simulink model "PassengerCar"  (R2019b)
settings: Solver=ode1  StartTime=0  StopTime=25  FixedStep=1.0000000000000000e-003  RelTol=1e-3
InitFcn:
  | sampleTime = str2double(get_param(bdroot, 'FixedStep'));
undefined symbols (not defined in the file or in its folder): AccPedalPos, BrakePedalPos, BrakeSwitch, DiscIntNeverNeededParam, DYNA4, EngSpd, IgnitionSwitch, InitialGear, InitialSpeed, IntendedEngTrq, LeftIndicator, MainBrakePress, MaxGear, MDL, MinGear, RefAcc, RefLane, RefLatPos, RefPath, RefPathCurv, RefSpd, RefSpdPreview, RefSpdRetrospect, RightIndicator, SteeringWheelAng, SteeringWheelTrq, UserDefinedRefValue, vm_const
libraries: UtilitiesLibrary x31, simulink x18, WheelSystemModules x13, LongitudinalControllerModules x13, LateralControllerModules x7, AnimationBusselectorModules x5, EnvironmentModules x5, BasicEngineControlModules x5, MiscellaneousControlModules x5, Animation3Modules x4, AuxiliariesModules x4, TireModules x4
(part 37 of 39)

== system PassengerCar/VehicleControl/LongitudinalControl/ControlSystemsPreprocessor/External Presetting of Controller /Presetting Source Identifiers ==
  note: SOURCE_NOMINALPATH = 1;
      | 	SOURCE_LANE = 2;
      | 	SOURCE_CONSTANT = 3;
      | 	SOURCE_TABLE_DISCRETE = 4;
      | 	SOURCE_TABLE_LINEAR = 5;
      | 	SOURCE_TABLE_CUBIC = 6;
      | 	SOURCE_TABLE_HAVERSINE = 7;
      | 	SOURCE_AUTOMATIC = 8;
      | 	SOURCE_SINE_TIME = 9;
      | 	SOURCE_SINE_PATH = 10;
      | 	SOURCE_HOLD = 11;
      | 	SOURCE_EXTERNAL = 12;
      | 	SOURCE_EXTERNAL_NOMINALPATH = 13;
      | 	SOURCE_EXTERNAL_LANE = 14;
  ExtCtrlVariablesEnforced : Inport
  SourceIdentifiers : Inport  Port=2
  Bus Selector : BusSelector  OutputSignals=CTRL_LongitudinalControl_RefSpdEnforced,CTRL_LongitudinalControl_RefAccEnforced,CTRL_LongitudinalControl_UserDefinedRefValueEnforced
  Bus Selector1 : BusSelector  OutputSignals=RefSpd,RefAcc,UserDefinedRefValue
  RefAccExternal : Constant  Value=vm_const('SOURCE_EXTERNAL')
  RefSpdExternal : Constant  Value=vm_const('SOURCE_EXTERNAL')
  SpeedCtrl_Spd : BusAssignment  AssignedSignals=RefSpd,RefSpdPreview,RefSpdRetrospect,RefAcc,UserDefinedRefValue
  Switch1 : Switch  Criteria=u2 > Threshold  OutDataTypeStr=Inherit: Inherit via back propagation
  Switch2 : Switch  Criteria=u2 > Threshold  OutDataTypeStr=Inherit: Inherit via back propagation
  Switch3 : Switch  Criteria=u2 > Threshold  OutDataTypeStr=Inherit: Inherit via back propagation
  UserDefinedRefValueExternal : Constant  Value=vm_const('SOURCE_EXTERNAL')
  ModifiedSourceIdentifiers : Outport  VectorParamsAs1DForOutWhenUnconnected=off
  wires:
  Bus Selector/3 -> Switch2/2  "<CTRL_LongitudinalControl_UserDefinedRefValueEnforced>"
  Bus Selector/1 -> Switch1/2  "<CTRL_LongitudinalControl_RefSpdEnforced>"
  Bus Selector/2 -> Switch3/2  "<CTRL_LongitudinalControl_RefAccEnforced>"
  Bus Selector1/3 -> Switch2/3  "<UserDefinedRefValue>"
  Bus Selector1/2 -> Switch3/3  "<RefAcc>"
  Switch3/1 -> SpeedCtrl_Spd/5
  RefAccExternal/1 -> Switch3/1
  Switch2/1 -> SpeedCtrl_Spd/6
  ExtCtrlVariablesEnforced/1 -> Bus Selector/1
  SourceIdentifiers/1 -> SpeedCtrl_Spd/1, Bus Selector1/1
  RefSpdExternal/1 -> Switch1/1
  Bus Selector1/1 -> Switch1/3  "<RefSpd>"
  UserDefinedRefValueExternal/1 -> Switch2/1
  Switch1/1 -> SpeedCtrl_Spd/4, SpeedCtrl_Spd/3, SpeedCtrl_Spd/2
  SpeedCtrl_Spd/1 -> ModifiedSourceIdentifiers/1

== system PassengerCar/VehicleControl/LongitudinalControl/ControlSystemsPreprocessor/External Presetting of Controller /Presetting Task Identifiers ==
  note: TASK_LONG_ACC_BRAKE_INPUTS = 1;
      | 	TASK_LONG_SPEED_CONTROL = 2;
      | 	TASK_LONG_ACCELERATION_CONTROL = 3;
      | 	TASK_LONG_USER_DEFINED = 4;
  ExtCtrlVariablesEnforced : Inport
  TaskIdentifiers : Inport  Port=2
  Bus Creator : BusCreator  Inputs=2
  Bus Selector : BusSelector  OutputSignals=CTRL_LongitudinalControl_RefSpdEnforced,CTRL_LongitudinalControl_RefAccEnforced,CTRL_LongitudinalControl_UserDefinedRefValueEnforced  OutputAsBus=on
  Bus Selector1 : BusSelector  OutputSignals=Task[-],Subtask[-]
  Bus to Vector : BusToVector
  Demux : Demux  Outputs=2
  Gain : Gain  Gain=[3 2 1]
  MinMax : MinMax  Function=max
  Multiport Switch : MultiPortSwitch  DataPortOrder=Zero-based contiguous  Inputs=4  zeroidx=on
  Mux : Mux  Inputs=2
  Speed Control : Constant  Value=[vm_const('TASK_LONG_SPEED_CONTROL') 0]
  Speed Control1 : Constant  Value=[vm_const('TASK_LONG_ACCELERATION_CONTROL') 0]
  Speed Control2 : Constant  Value=[vm_const('TASK_LONG_USER_DEFINED') 0]
  ModifiedTaskIdentifiers : Outport  VectorParamsAs1DForOutWhenUnconnected=off
  wires:
  Speed Control1/1 -> Multiport Switch/4
  Speed Control2/1 -> Multiport Switch/3
  Speed Control/1 -> Multiport Switch/5
  Bus Creator/1 -> ModifiedTaskIdentifiers/1
  ExtCtrlVariablesEnforced/1 -> Bus Selector/1
  Demux/2 -> Bus Creator/2  "Subtask"
  Demux/1 -> Bus Creator/1  "Task"
  Multiport Switch/1 -> Demux/1
  TaskIdentifiers/1 -> Bus Selector1/1
  Bus Selector1/1 -> Mux/1  "<Task[-]>"
  Bus Selector1/2 -> Mux/2  "<Subtask[-]>"
  Gain/1 -> MinMax/1
  Bus to Vector/1 -> Gain/1
  Bus Selector/1 -> Bus to Vector/1
  MinMax/1 -> Multiport Switch/1
  Mux/1 -> Multiport Switch/2

== system PassengerCar/VehicleControl/LongitudinalControl/ControlSystemsPreprocessor/Generation of Hold Data/DefaultAction Subsystem ==
  HoldData : Inport
  Action Port : ActionPort  InitializeStates=reset  ActionPortLabel=default:
  HoldLongitudinalControlInputs : Outport  VectorParamsAs1DForOutWhenUnconnected=off
  wires:
  HoldData/1 -> HoldLongitudinalControlInputs/1

== system PassengerCar/VehicleControl/LongitudinalControl/ControlSystemsPreprocessor/Generation of Hold Data/Enabled Subsystem ==
  LongCTRL : Inport
  VehicleInfo : Inport  Port=2
  Enable : EnablePort  StatesWhenEnabling=reset  PropagateVarSize=During execution
  Add : Sum  Inputs=+-
  All zeros TD_BO_LongitudinalControlInputs : Constant  Value=0  OutDataTypeStr=Bus: TD_BO_LongitudinalControlInputs
  Bus Assignment : BusAssignment  AssignedSignals=AccPedalPos,BrakePedalPos,MainBrakePress,FrontLeftWheelBrakePress,FrontRightWheelBrakePress,RearLeftWheelBrakePress,RearRightWheelBrakePress,Rear2LeftWheelBrakePress,Rear2RightWheelBrakePress,Rear3LeftWheelBrakePress,Rear3RightWheelBrakePress,TrailerFrontLeftWheelBrakePress,TrailerFrontRightWheelBrakePress,TrailerRearLeftWheelBrakePress,TrailerRearRightWheelBrakePress,TrailerRear2LeftWheelBrakePress,TrailerRear2RightWheelBrakePress,TrailerRear3LeftWheelBrakePress,TrailerRear3RightWheelBrakePress,MinGear,MaxGear,ClutchPedalPos,ShiftingProgramSelection,IgnitionSwitch,Handbrake,ParkingLock,FrontDifferentialLock,RearDifferentialLock,Rear2DifferentialLock,Rear3DifferentialLock,TransferCaseLock,DayRunningLight,LowBeamLight,HighBeamLight,FogLampFront,FogLampRear,ESCSwitch,ABSSwitch,ACCSwitch,ACCRefSpd,AEBSwitch,RefSpd,RefSpdPreview,RefSpdRetrospect,RefAcc
  Bus Selector1 : BusSelector  OutputSignals=Chassis_VehicleBody_AbsVel[m/s],Chassis_VehicleBody_Acc_wrt_WorldSys(VehSys)[m/s**2]
  Bus Selector15 : BusSelector  OutputSignals=AccPedalPos[0_1],BrakePedalPos[0_1],MainBrakePress[Pa],FrontLeftWheelBrakePress[Pa],FrontRightWheelBrakePress[Pa],RearLeftWheelBrakePress[Pa],RearRightWheelBrakePress[Pa],Rear2LeftWheelBrakePress[Pa],Rear2RightWheelBrakePress[Pa],Rear3LeftWheelBrakePress[Pa],Rear3RightWheelBrakePress[Pa],TrailerFrontLeftWheelBrakePress[Pa],TrailerFrontRightWheelBrakePress[Pa],TrailerRearLeftWheelBrakePress[Pa],TrailerRearRightWheelBrakePress[Pa],TrailerRear2LeftWheelBrakePress[Pa],TrailerRear2RightWheelBrakePress[Pa],TrailerRear3LeftWheelBrakePress[Pa],TrailerRear3RightWheelBrakePress[Pa],MinGear[-4;20],MaxGear[-4;20],ClutchPos[0_1],ShiftingProgramSelection[-],IgnitionSwitch[0;3],Handbrake[0_1],ParkingLock[0;1],FrontDifferentialLock[0;1],RearDifferentialLock[0;1],Rear2DifferentialLock[0;1],Rear3DifferentialLock[0;1],TransferCaseLock[0;1],DayRunningLight[0;1],LowBeamLight[0;1],HighBeamLight[0;1],FogLampFront[0;1],FogLampRear[0;1],ESCSwitch[0;1],ABSSwitch[0;1],ACCSwitch[0;1],ACCRefSpd[m/s],AEBSwitch[0;1]
  Constant1 : Constant
  y component : Selector  InputPortWidth=3  IndexOptions=Index vector (dialog)  Indices=1  OutputSizes=1
  HoldData : Outport  VectorParamsAs1DForOutWhenUnconnected=off
  wires:
  Bus Selector15/21 -> Bus Assignment/22  "<MaxGear[-4;20]>"
  Bus Selector15/20 -> Bus Assignment/21  "<MinGear[-4;20]>"
  Bus Selector15/22 -> Add/2  "<ClutchPos[0_1]>"
  Bus Selector15/29 -> Bus Assignment/30  "<Rear2DifferentialLock[0;1]>"
  Bus Selector15/31 -> Bus Assignment/32  "<TransferCaseLock[0;1]>"
  Bus Selector15/6 -> Bus Assignment/7  "<RearLeftWheelBrakePress[Pa]>"
  Bus Selector15/28 -> Bus Assignment/29  "<RearDifferentialLock[0;1]>"
  Bus Selector15/17 -> Bus Assignment/18  "<TrailerRear2RightWheelBrakePress[Pa]>"
  Bus Selector15/36 -> Bus Assignment/37  "<FogLampRear[0;1]>"
  Bus Selector15/30 -> Bus Assignment/31  "<Rear3DifferentialLock[0;1]>"
  Bus Selector15/13 -> Bus Assignment/14  "<TrailerFrontRightWheelBrakePress[Pa]>"
  Bus Selector15/35 -> Bus Assignment/36  "<FogLampFront[0;1]>"
  Bus Selector15/2 -> Bus Assignment/3  "<BrakePedalPos[0_1]>"
  Bus Selector15/16 -> Bus Assignment/17  "<TrailerRear2LeftWheelBrakePress[Pa]>"
  Bus Selector15/15 -> Bus Assignment/16  "<TrailerRearRightWheelBrakePress[Pa]>"
  Bus Selector15/9 -> Bus Assignment/10  "<Rear2RightWheelBrakePress[Pa]>"
  Bus Selector15/19 -> Bus Assignment/20  "<TrailerRear3RightWheelBrakePress[Pa]>"
  Bus Selector15/23 -> Bus Assignment/24  "<ShiftingProgramSelection[-]>"
  Bus Selector15/8 -> Bus Assignment/9  "<Rear2LeftWheelBrakePress[Pa]>"
  Bus Selector15/34 -> Bus Assignment/35  "<HighBeamLight[0;1]>"
  Bus Selector15/24 -> Bus Assignment/25  "<IgnitionSwitch[0;3]>"
  Bus Selector15/33 -> Bus Assignment/34  "<LowBeamLight[0;1]>"
  Bus Selector15/26 -> Bus Assignment/27  "<ParkingLock[0;1]>"
  Bus Selector15/25 -> Bus Assignment/26  "<Handbrake[0_1]>"
  Bus Selector15/12 -> Bus Assignment/13  "<TrailerFrontLeftWheelBrakePress[Pa]>"
  Bus Selector15/10 -> Bus Assignment/11  "<Rear3LeftWheelBrakePress[Pa]>"
  Bus Selector15/14 -> Bus Assignment/15  "<TrailerRearLeftWheelBrakePress[Pa]>"
  Bus Selector15/7 -> Bus Assignment/8  "<RearRightWheelBrakePress[Pa]>"
  Bus Selector15/5 -> Bus Assignment/6  "<FrontRightWheelBrakePress[Pa]>"
  Bus Selector15/1 -> Bus Assignment/2  "<AccPedalPos[0_1]>"
  Bus Selector15/32 -> Bus Assignment/33  "<DayRunningLight[0;1]>"
  Bus Selector15/11 -> Bus Assignment/12  "<Rear3RightWheelBrakePress[Pa]>"
  Bus Selector15/3 -> Bus Assignment/4  "<MainBrakePress[Pa]>"
  Bus Selector15/27 -> Bus Assignment/28  "<FrontDifferentialLock[0;1]>"
  Bus Selector15/4 -> Bus Assignment/5  "<FrontLeftWheelBrakePress[Pa]>"
  Bus Selector15/18 -> Bus Assignment/19  "<TrailerRear3LeftWheelBrakePress[Pa]>"
  Bus Selector15/39 -> Bus Assignment/40  "<ACCSwitch[0;1]>"
  Bus Selector15/37 -> Bus Assignment/38  "<ESCSwitch[0;1]>"
  Bus Selector15/38 -> Bus Assignment/39  "<ABSSwitch[0;1]>"
  All zeros TD_BO_LongitudinalControlInputs/1 -> Bus Assignment/1
  Bus Selector15/40 -> Bus Assignment/41  "<ACCRefSpd[m/s]>"
  Bus Selector15/41 -> Bus Assignment/42  "<AEBSwitch[0;1]>"
  Bus Selector1/2 -> y component/1  "<Chassis_VehicleBody_Acc_wrt_WorldSys(VehSys)[m/s**2]>"
  Constant1/1 -> Add/1
  y component/1 -> Bus Assignment/46  "RefAcc"
  LongCTRL/1 -> Bus Selector15/1
  VehicleInfo/1 -> Bus Selector1/1
  Bus Assignment/1 -> HoldData/1
  Add/1 -> Bus Assignment/23  "ClutchPedalPos[0_1]"
  Bus Selector1/1 -> Bus Assignment/45, Bus Assignment/44, Bus Assignment/43  "<Chassis_VehicleBody_AbsVel[m/s]>"

== system PassengerCar/VehicleControl/LongitudinalControl/ControlSystemsPreprocessor/Generation of Hold Data/InitialAction Subsystem ==
  LongitudinalControlInputs : Inport
  Action Port : ActionPort  InitializeStates=reset  ActionPortLabel=case [ 1 ]:
  All zeros TD_BO_LongitudinalControlInputs : Constant  Value=0  OutDataTypeStr=Bus: TD_BO_LongitudinalControlInputs
  Bus Assignment : BusAssignment  AssignedSignals=InitialSpeed,RefSpd,RefSpdPreview,RefSpdRetrospect,InitialGear,MinGear,MaxGear
  Bus Selector1 : BusSelector  OutputSignals=InitialSpeed,InitialGear
  InitialLongitudinalControlInputs : Outport  VectorParamsAs1DForOutWhenUnconnected=off
  wires:
  Bus Selector1/2 -> Bus Assignment/6, Bus Assignment/7, Bus Assignment/8  "<InitialGear>"
  All zeros TD_BO_LongitudinalControlInputs/1 -> Bus Assignment/1
  Bus Selector1/1 -> Bus Assignment/5, Bus Assignment/4, Bus Assignment/3, Bus Assignment/2  "<InitialSpeed>"
  Bus Assignment/1 -> InitialLongitudinalControlInputs/1
  LongitudinalControlInputs/1 -> Bus Selector1/1

== system PassengerCar/VehicleControl/LongitudinalControl/ControlSystemsPreprocessor/Generation of Speed Data/Smooth Derivative ==
  note: This transfer function calculates a smooth acceleration with continuous jerk from a speed input signal.
      | The smoothing time constant T = previewTime / 2 is an input signal.
  RefSpdPrev[m/s] : Inport
  PreviewTime[s] : Inport  Port=2
  Enable : EnablePort  StatesWhenEnabling=reset
  Gain1 : Gain  Gain=0.5
  Max : MinMax  Function=max  Inputs=2
  Transfer Fcn with variable prameter : Subsystem
      mask Display: disp('num = s \n den = T^2*s^2 + 2*T*s + 1')
  limit to +/-20 : Saturate  UpperLimit=20  LowerLimit=-20
  minimum smoothing constant : Constant  Value=0.01
  SmoothedRefAcc[m/s**2] : Outport  OutputWhenDisabled=reset  InitialOutput=0  VectorParamsAs1DForOutWhenUnconnected=off
  wires:
  PreviewTime[s]/1 -> Gain1/1
  minimum smoothing constant/1 -> Max/2
  Gain1/1 -> Max/1
  RefSpdPrev[m/s]/1 -> Transfer Fcn with variable prameter/1(u)
  Max/1 -> Transfer Fcn with variable prameter/2(T)
  Transfer Fcn with variable prameter/1(y) -> limit to +/-20/1
  limit to +/-20/1 -> SmoothedRefAcc[m/s**2]/1

== system PassengerCar/VehicleControl/LongitudinalControl/ControlSystemsPreprocessor/Generation of Speed Data/Target Speed Computation Check ==
  note: TASK_LONG_ACC_BRAKE_INPUTS = 1;
      | TASK_LONG_SPEED_CONTROL = 2;
      | TASK_LONG_ACCELERATION_CONTROL = 3;
      | TASK_LONG_USER_DEFINED = 4;
  note: SOURCE_NOMINALPATH = 1;
      | 	SOURCE_LANE = 2;
      | 	SOURCE_CONSTANT = 3;
      | 	SOURCE_TABLE_DISCRETE = 4;
      | 	SOURCE_TABLE_LINEAR = 5;
      | 	SOURCE_TABLE_CUBIC = 6;
      | 	SOURCE_TABLE_HAVERSINE = 7;
      | 	SOURCE_AUTOMATIC = 8;
      | 	SOURCE_SINE_TIME = 9;
      | 	SOURCE_SINE_PATH = 10;
      | 	SOURCE_HOLD = 11;
      | 	SOURCE_EXTERNAL = 12;
      | 	SOURCE_EXTERNAL_NOMINALPATH = 13;
      | 	SOURCE_EXTERNAL_LANE = 14;
  TaskIdentifiers : Inport
  SourceIdentifiers : Inport  Port=2
  Bus Selector : BusSelector  OutputSignals=RefSpd
  Bus Selector1 : BusSelector  OutputSignals=Task
  Compare To Constant : simulink/Logic and Bit Operations/Compare To Constant  relop===  const=vm_const('TASK_LONG_SPEED_CONTROL')  OutDataTypeStr=boolean  ZeroCross=off
  Compare To Constant1 : simulink/Logic and Bit Operations/Compare To Constant  relop===  const=vm_const('SOURCE_AUTOMATIC')  OutDataTypeStr=uint8  ZeroCross=off
  Compare To Constant2 : simulink/Logic and Bit Operations/Compare To Constant  relop===  const=vm_const('TASK_LONG_USER_DEFINED')  OutDataTypeStr=boolean  ZeroCross=off
  Compare To Constant3 : simulink/Logic and Bit Operations/Compare To Constant  relop===  const=vm_const('TASK_LONG_ACCELERATION_CONTROL')  OutDataTypeStr=boolean  ZeroCross=off
  Data Type Conversion : DataTypeConversion  OutDataTypeStr=int8
  Logical Operator : Logic  AllPortsSameDT=off
  Logical Operator1 : Logic  Operator=OR  AllPortsSameDT=off
  Logical Operator3 : Logic  AllPortsSameDT=off
  Logical Operator4 : Logic  Operator=NOT  AllPortsSameDT=off
  isAutomatic : Outport  VectorParamsAs1DForOutWhenUnconnected=off
  isAccelerationControl : Outport  Port=2  VectorParamsAs1DForOutWhenUnconnected=off
  needsSmoothedDerivative : Outport  Port=3  VectorParamsAs1DForOutWhenUnconnected=off
  wires:
  Compare To Constant3/1 -> isAccelerationControl/1
  Data Type Conversion/1 -> Compare To Constant1/1
  Logical Operator1/1 -> Logical Operator/1
  Compare To Constant/1 -> Logical Operator3/1, Logical Operator1/1
  Compare To Constant2/1 -> Logical Operator1/2
  Logical Operator/1 -> isAutomatic/1
  Compare To Constant1/1 -> Logical Operator4/1, Logical Operator/2
  SourceIdentifiers/1 -> Bus Selector/1
  Bus Selector/1 -> Data Type Conversion/1  "<RefSpd>"
  Bus Selector1/1 -> Compare To Constant2/1, Compare To Constant/1, Compare To Constant3/1  "<Task>"
  TaskIdentifiers/1 -> Bus Selector1/1
  Logical Operator4/1 -> Logical Operator3/2
  Logical Operator3/1 -> needsSmoothedDerivative/1

== system PassengerCar/Vehicle/BrakeSystem/BrakeSystemControlUnit/BasicElectronicStabilityControl/BasicAntiLockBrakeControl/AntiLockBrakeSystemOutput ==
  FrontLeftWheelBrakeControllerState[0;3]___UNIQUE_1 : Inport  Description=|  PortDimensions=[1]
      | <name>FrontLeftWheelBrakeControllerState[0;3]</name>
      | <comment></comment>
  FrontRightWheelBrakeControllerState[0;3]___UNIQUE_1 : Inport  Description=|  Port=2  PortDimensions=[1]
      | <name>FrontRightWheelBrakeControllerState[0;3]</name>
      | <comment></comment>
  RearLeftWheelBrakeControllerState[0;3]___UNIQUE_1 : Inport  Description=|  Port=3  PortDimensions=[1]
      | <name>RearLeftWheelBrakeControllerState[0;3]</name>
      | <comment></comment>
  RearRightWheelBrakeControllerState[0;3]___UNIQUE_1 : Inport  Description=|  Port=4  PortDimensions=[1]
      | <name>RearRightWheelBrakeControllerState[0;3]</name>
      | <comment></comment>
  FrontLeftAntiLockBrakeSystemActive[0;1]___UNIQUE_1 : Inport  Description=|  Port=5  PortDimensions=[1]
      | <name>FrontLeftAntiLockBrakeSystemActive[0;1]</name>
      | <comment></comment>
  FrontRightAntiLockBrakeSystemActive[0;1]___UNIQUE_1 : Inport  Description=|  Port=6  PortDimensions=[1]
      | <name>FrontRightAntiLockBrakeSystemActive[0;1]</name>
      | <comment></comment>
  RearLeftAntiLockBrakeSystemActive[0;1]___UNIQUE_1 : Inport  Description=|  Port=7  PortDimensions=[1]
      | <name>RearLeftAntiLockBrakeSystemActive[0;1]</name>
      | <comment></comment>
  RearRightAntiLockBrakeSystemActive[0;1]___UNIQUE_1 : Inport  Description=|  Port=8  PortDimensions=[1]
      | <name>RearRightAntiLockBrakeSystemActive[0;1]</name>
      | <comment></comment>
  Enabled[0;1]___UNIQUE_1 : Inport  Description=|  Port=9  PortDimensions=[1]
      | <name>Enabled[0;1]</name>
      | <comment></comment>
  Active[0;1]___UNIQUE_1 : Inport  Description=|  Port=10  PortDimensions=[1]
      | <name>Active[0;1]</name>
      | <comment></comment>
  __TDD__AntiLockBrakeSystemInfo.Active[0;1] : Demux  Outputs=[1]
  __TDD__AntiLockBrakeSystemInfo.Enabled[0;1] : Demux  Outputs=[1]
  __TDD__AntiLockBrakeSystemInfo.FrontLeft.AntiLockBrakeSystemActive[0;1] : Demux  Outputs=[1]
  __TDD__AntiLockBrakeSystemInfo.FrontLeft.WheelBrakeControllerState[0;3] : Demux  Outputs=[1]
  __TDD__AntiLockBrakeSystemInfo.FrontRight.AntiLockBrakeSystemActive[0;1] : Demux  Outputs=[1]
  __TDD__AntiLockBrakeSystemInfo.FrontRight.WheelBrakeControllerState[0;3] : Demux  Outputs=[1]
  __TDD__AntiLockBrakeSystemInfo.RearLeft.AntiLockBrakeSystemActive[0;1] : Demux  Outputs=[1]
  __TDD__AntiLockBrakeSystemInfo.RearLeft.WheelBrakeControllerState[0;3] : Demux  Outputs=[1]
  __TDD__AntiLockBrakeSystemInfo.RearRight.AntiLockBrakeSystemActive[0;1] : Demux  Outputs=[1]
  __TDD__AntiLockBrakeSystemInfo.RearRight.WheelBrakeControllerState[0;3] : Demux  Outputs=[1]
  __TDO__AntiLockBrakeSystemInfo : BusCreator  Inputs=6
  __TDO__AntiLockBrakeSystemInfo.FrontLeft : BusCreator  Inputs=2
  __TDO__AntiLockBrakeSystemInfo.FrontRight : BusCreator  Inputs=2
  __TDO__AntiLockBrakeSystemInfo.RearLeft : BusCreator  Inputs=2
  __TDO__AntiLockBrakeSystemInfo.RearRight : BusCreator  Inputs=2
  AntiLockBrakeSystemInfo___UNIQUE_1 : Outport  Description=|  PortDimensions=[10]  VectorParamsAs1DForOutWhenUnconnected=off
      | <name>FrontLeftWheelBrakeControllerState[0;3]</name>
      | <comment></comment>
  wires:
  FrontLeftWheelBrakeControllerState[0;3]___UNIQUE_1/1 -> __TDD__AntiLockBrakeSystemInfo.FrontLeft.WheelBrakeControllerState[0;3]/1
  __TDD__AntiLockBrakeSystemInfo.FrontLeft.WheelBrakeControllerState[0;3]/1 -> __TDO__AntiLockBrakeSystemInfo.FrontLeft/1  "WheelBrakeControllerState[0;3]"
  __TDO__AntiLockBrakeSystemInfo.FrontLeft/1 -> __TDO__AntiLockBrakeSystemInfo/1  "FrontLeft"
  FrontRightWheelBrakeControllerState[0;3]___UNIQUE_1/1 -> __TDD__AntiLockBrakeSystemInfo.FrontRight.WheelBrakeControllerState[0;3]/1
  __TDD__AntiLockBrakeSystemInfo.FrontRight.WheelBrakeControllerState[0;3]/1 -> __TDO__AntiLockBrakeSystemInfo.FrontRight/1  "WheelBrakeControllerState[0;3]"
  __TDO__AntiLockBrakeSystemInfo.FrontRight/1 -> __TDO__AntiLockBrakeSystemInfo/2  "FrontRight"
  RearLeftWheelBrakeControllerState[0;3]___UNIQUE_1/1 -> __TDD__AntiLockBrakeSystemInfo.RearLeft.WheelBrakeControllerState[0;3]/1
  __TDD__AntiLockBrakeSystemInfo.RearLeft.WheelBrakeControllerState[0;3]/1 -> __TDO__AntiLockBrakeSystemInfo.RearLeft/1  "WheelBrakeControllerState[0;3]"
  __TDO__AntiLockBrakeSystemInfo.RearLeft/1 -> __TDO__AntiLockBrakeSystemInfo/3  "RearLeft"
  RearRightWheelBrakeControllerState[0;3]___UNIQUE_1/1 -> __TDD__AntiLockBrakeSystemInfo.RearRight.WheelBrakeControllerState[0;3]/1
  __TDD__AntiLockBrakeSystemInfo.RearRight.WheelBrakeControllerState[0;3]/1 -> __TDO__AntiLockBrakeSystemInfo.RearRight/1  "WheelBrakeControllerState[0;3]"
  __TDO__AntiLockBrakeSystemInfo.RearRight/1 -> __TDO__AntiLockBrakeSystemInfo/4  "RearRight"
  FrontLeftAntiLockBrakeSystemActive[0;1]___UNIQUE_1/1 -> __TDD__AntiLockBrakeSystemInfo.FrontLeft.AntiLockBrakeSystemActive[0;1]/1
  __TDD__AntiLockBrakeSystemInfo.FrontLeft.AntiLockBrakeSystemActive[0;1]/1 -> __TDO__AntiLockBrakeSystemInfo.FrontLeft/2  "AntiLockBrakeSystemActive[0;1]"
  FrontRightAntiLockBrakeSystemActive[0;1]___UNIQUE_1/1 -> __TDD__AntiLockBrakeSystemInfo.FrontRight.AntiLockBrakeSystemActive[0;1]/1
  __TDD__AntiLockBrakeSystemInfo.FrontRight.AntiLockBrakeSystemActive[0;1]/1 -> __TDO__AntiLockBrakeSystemInfo.FrontRight/2  "AntiLockBrakeSystemActive[0;1]"
  RearLeftAntiLockBrakeSystemActive[0;1]___UNIQUE_1/1 -> __TDD__AntiLockBrakeSystemInfo.RearLeft.AntiLockBrakeSystemActive[0;1]/1
  __TDD__AntiLockBrakeSystemInfo.RearLeft.AntiLockBrakeSystemActive[0;1]/1 -> __TDO__AntiLockBrakeSystemInfo.RearLeft/2  "AntiLockBrakeSystemActive[0;1]"
  RearRightAntiLockBrakeSystemActive[0;1]___UNIQUE_1/1 -> __TDD__AntiLockBrakeSystemInfo.RearRight.AntiLockBrakeSystemActive[0;1]/1
  __TDD__AntiLockBrakeSystemInfo.RearRight.AntiLockBrakeSystemActive[0;1]/1 -> __TDO__AntiLockBrakeSystemInfo.RearRight/2  "AntiLockBrakeSystemActive[0;1]"
  Enabled[0;1]___UNIQUE_1/1 -> __TDD__AntiLockBrakeSystemInfo.Enabled[0;1]/1
  __TDD__AntiLockBrakeSystemInfo.Enabled[0;1]/1 -> __TDO__AntiLockBrakeSystemInfo/5  "Enabled[0;1]"
  Active[0;1]___UNIQUE_1/1 -> __TDD__AntiLockBrakeSystemInfo.Active[0;1]/1
  __TDD__AntiLockBrakeSystemInfo.Active[0;1]/1 -> __TDO__AntiLockBrakeSystemInfo/6  "Active[0;1]"
  __TDO__AntiLockBrakeSystemInfo/1 -> AntiLockBrakeSystemInfo___UNIQUE_1/1  "AntiLockBrakeSystemInfo"

== system PassengerCar/Vehicle/BrakeSystem/BrakeSystemControlUnit/BasicElectronicStabilityControl/BasicYawStabilityControl/PrepareBrakeTrqPressRatioInput ==
  note: Memory block in place to avoid
      | 'Algebraic loop' error in Simulink
  FrontBrakeTrqPressRatio[m**3] : Inport
  RearBrakeTrqPressRatio[m**3] : Inport  Port=2
  Add : Sum
  Constant1 : Constant  Value=2
  Divide : Product  Inputs=*/
  Memory : Memory  InheritSampleTime=on
  AverageBrakeTrqPressRatio[m**3] : Outport  VectorParamsAs1DForOutWhenUnconnected=off
  wires:
  Memory/1 -> Divide/1
  Add/1 -> Memory/1
  RearBrakeTrqPressRatio[m**3]/1 -> Add/2
  Divide/1 -> AverageBrakeTrqPressRatio[m**3]/1
  Constant1/1 -> Divide/2
  FrontBrakeTrqPressRatio[m**3]/1 -> Add/1

== system PassengerCar/Vehicle/BrakeSystem/BrakeSystemControlUnit/BasicElectronicStabilityControl/BasicYawStabilityControl/PrepareTireRadiusInput ==
  FrontLeftTireRadius[m] : Inport
  RearLeftTireRadius[m] : Inport  Port=2
  Add : Sum
  Constant1 : Constant  Value=2
  Divide : Product  Inputs=*/
  AverageTireRadius[m] : Outport  VectorParamsAs1DForOutWhenUnconnected=off
  wires:
  RearLeftTireRadius[m]/1 -> Add/2
  FrontLeftTireRadius[m]/1 -> Add/1
  Constant1/1 -> Divide/2
  Add/1 -> Divide/1
  Divide/1 -> AverageTireRadius[m]/1

== system PassengerCar/Vehicle/BrakeSystem/BrakeSystemControlUnit/BasicElectronicStabilityControl/BasicYawStabilityControl/PrepareWheelTrackInput ==
  FrontWheelTrack[m] : Inport
  RearWheelTrack[m] : Inport  Port=2
  Add : Sum
  Constant1 : Constant  Value=2
  Divide : Product  Inputs=*/
  AverageWheelTrack[m] : Outport  VectorParamsAs1DForOutWhenUnconnected=off
  wires:
  Divide/1 -> AverageWheelTrack[m]/1
  RearWheelTrack[m]/1 -> Add/2
  FrontWheelTrack[m]/1 -> Add/1
  Constant1/1 -> Divide/2
  Add/1 -> Divide/1

== system PassengerCar/Vehicle/BrakeSystem/BrakeSystemControlUnit/BasicElectronicStabilityControl/BasicYawStabilityControl/YawStabilityControlOutput ==
  Active[0;1]___UNIQUE_1 : Inport  Description=|  PortDimensions=[1]
      | <name>Active[0;1]</name>
      | <comment></comment>
  Enabled[0;1]___UNIQUE_1 : Inport  Description=|  Port=2  PortDimensions=[1]
      | <name>Enabled[0;1]</name>
      | <comment></comment>
  __TDD__YawStabilityControlInfo.Active[0;1] : Demux  Outputs=[1]
  __TDD__YawStabilityControlInfo.Enabled[0;1] : Demux  Outputs=[1]
  __TDO__YawStabilityControlInfo : BusCreator  Inputs=2
  YawStabilityControlInfo___UNIQUE_1 : Outport  Description=|  PortDimensions=[2]  VectorParamsAs1DForOutWhenUnconnected=off
      | <name>Active[0;1]</name>
      | <comment></comment>
  wires:
  Active[0;1]___UNIQUE_1/1 -> __TDD__YawStabilityControlInfo.Active[0;1]/1
  __TDD__YawStabilityControlInfo.Active[0;1]/1 -> __TDO__YawStabilityControlInfo/1  "Active[0;1]"
  Enabled[0;1]___UNIQUE_1/1 -> __TDD__YawStabilityControlInfo.Enabled[0;1]/1
  __TDD__YawStabilityControlInfo.Enabled[0;1]/1 -> __TDO__YawStabilityControlInfo/2  "Enabled[0;1]"
  __TDO__YawStabilityControlInfo/1 -> YawStabilityControlInfo___UNIQUE_1/1  "YawStabilityControlInfo"

== system PassengerCar/Vehicle/Drivetrain/DrivetrainPhysics/DrivetrainPhysicsOutputs/ClutchOutput/ClutchOutput ==
  Trq[Nm]___UNIQUE_1 : Inport  Description=|  PortDimensions=[1]
      | <name>Trq[Nm]</name>
      | <comment></comment>
  Pos[0_1]___UNIQUE_1 : Inport  Description=|  Port=2  PortDimensions=[1]
      | <name>Pos[0_1]</name>
      | <comment></comment>
  __TDD__Clutch.Pos[0_1] : Demux  Outputs=[1]
  __TDD__Clutch.Trq[Nm] : Demux  Outputs=[1]
  __TDO__Clutch : BusCreator  Inputs=2
  Clutch___UNIQUE_1 : Outport  Description=|  PortDimensions=[2]  VectorParamsAs1DForOutWhenUnconnected=off
      | <name>Trq[Nm]</name>
      | <comment></comment>
  wires:
  Trq[Nm]___UNIQUE_1/1 -> __TDD__Clutch.Trq[Nm]/1
  __TDD__Clutch.Trq[Nm]/1 -> __TDO__Clutch/1  "Trq[Nm]"
  Pos[0_1]___UNIQUE_1/1 -> __TDD__Clutch.Pos[0_1]/1
  __TDD__Clutch.Pos[0_1]/1 -> __TDO__Clutch/2  "Pos[0_1]"
  __TDO__Clutch/1 -> Clutch___UNIQUE_1/1  "Clutch"

== system PassengerCar/Vehicle/Drivetrain/DrivetrainPhysics/DrivetrainPhysicsOutputs/FrontDifferentialOutput/FrontDifferentialOutput ==
  InSpd[rad/s]___UNIQUE_1 : Inport  Description=|  PortDimensions=[1]
      | <name>InSpd[rad/s]</name>
      | <comment></comment>
  LeftOutCutTrq[Nm]___UNIQUE_1 : Inport  Description=|  Port=2  PortDimensions=[1]
      | <name>LeftOutCutTrq[Nm]</name>
      | <comment></comment>
  RightOutCutTrq[Nm]___UNIQUE_1 : Inport  Description=|  Port=3  PortDimensions=[1]
      | <name>RightOutCutTrq[Nm]</name>
      | <comment></comment>
  LossPower[W]___UNIQUE_1 : Inport  Description=|  Port=4  PortDimensions=[1]
      | <name>LossPower[W]</name>
      | <comment></comment>
  __TDD__FrontDifferential.InSpd[rad/s] : Demux  Outputs=[1]
  __TDD__FrontDifferential.LeftOutCutTrq[Nm] : Demux  Outputs=[1]
  __TDD__FrontDifferential.LossPower[W] : Demux  Outputs=[1]
  __TDD__FrontDifferential.RightOutCutTrq[Nm] : Demux  Outputs=[1]
  __TDO__FrontDifferential : BusCreator  Inputs=4
  FrontDifferential___UNIQUE_1 : Outport  Description=|  PortDimensions=[4]  VectorParamsAs1DForOutWhenUnconnected=off
      | <name>InSpd[rad/s]</name>
      | <comment></comment>
  wires:
  InSpd[rad/s]___UNIQUE_1/1 -> __TDD__FrontDifferential.InSpd[rad/s]/1
  __TDD__FrontDifferential.InSpd[rad/s]/1 -> __TDO__FrontDifferential/1  "InSpd[rad/s]"
  LeftOutCutTrq[Nm]___UNIQUE_1/1 -> __TDD__FrontDifferential.LeftOutCutTrq[Nm]/1
  __TDD__FrontDifferential.LeftOutCutTrq[Nm]/1 -> __TDO__FrontDifferential/2  "LeftOutCutTrq[Nm]"
  RightOutCutTrq[Nm]___UNIQUE_1/1 -> __TDD__FrontDifferential.RightOutCutTrq[Nm]/1
  __TDD__FrontDifferential.RightOutCutTrq[Nm]/1 -> __TDO__FrontDifferential/3  "RightOutCutTrq[Nm]"
  LossPower[W]___UNIQUE_1/1 -> __TDD__FrontDifferential.LossPower[W]/1
  __TDD__FrontDifferential.LossPower[W]/1 -> __TDO__FrontDifferential/4  "LossPower[W]"
  __TDO__FrontDifferential/1 -> FrontDifferential___UNIQUE_1/1  "FrontDifferential"

== system PassengerCar/Vehicle/Drivetrain/DrivetrainPhysics/DrivetrainPhysicsOutputs/FrontLeftShaftOutput/FrontLeftShaftOutput ==
  Trq[Nm]___UNIQUE_1 : Inport  Description=|  PortDimensions=[1]
      | <name>Trq[Nm]</name>
      | <comment></comment>
  RotSpdDifferentialOut[rad/s]___UNIQUE_1 : Inport  Description=|  Port=2  PortDimensions=[1]
      | <name>RotSpdDifferentialOut[rad/s]</name>
      | <comment></comment>
  RotAcc[rad/s**2]___UNIQUE_1 : Inport  Description=|  Port=3  PortDimensions=[1]
      | <name>RotAcc[rad/s**2]</name>
      | <comment></comment>
  DerivativeOfTrq_wrt_RotAng[Nm/rad]___UNIQUE_1 : Inport  Description=|  Port=4  PortDimensions=[1]
      | <name>DerivativeOfTrq_wrt_RotAng[Nm/rad]</name>
      | <comment></comment>
  DerivativeOfTrq_wrt_WheelSpd[Nm/(rad/s)]___UNIQUE_1 : Inport  Description=|  Port=5  PortDimensions=[1]
      | <name>DerivativeOfTrq_wrt_WheelSpd[Nm/(rad/s)]</name>
      | <comment></comment>
  AddInrt[kg*m**2]___UNIQUE_1 : Inport  Description=|  Port=6  PortDimensions=[1]
      | <name>AddInrt[kg*m**2]</name>
      | <comment></comment>
  FrictionTrq[Nm]___UNIQUE_1 : Inport  Description=|  Port=7  PortDimensions=[1]
      | <name>FrictionTrq[Nm]</name>
      | <comment></comment>
  __TDD__FrontLeftShaft.AddInrt[kg*m**2] : Demux  Outputs=[1]
  __TDD__FrontLeftShaft.DerivativeOfTrq_wrt_RotAng[Nm/rad] : Demux  Outputs=[1]
  __TDD__FrontLeftShaft.DerivativeOfTrq_wrt_WheelSpd[Nm/(rad/s)] : Demux  Outputs=[1]
  __TDD__FrontLeftShaft.FrictionTrq[Nm] : Demux  Outputs=[1]
  __TDD__FrontLeftShaft.RotAcc[rad/s**2] : Demux  Outputs=[1]
  __TDD__FrontLeftShaft.RotSpdDifferentialOut[rad/s] : Demux  Outputs=[1]
  __TDD__FrontLeftShaft.Trq[Nm] : Demux  Outputs=[1]
  __TDO__FrontLeftShaft : BusCreator  Inputs=7
  FrontLeftShaft___UNIQUE_1 : Outport  Description=|  PortDimensions=[7]  VectorParamsAs1DForOutWhenUnconnected=off
      | <name>Trq[Nm]</name>
      | <comment></comment>
  wires:
  Trq[Nm]___UNIQUE_1/1 -> __TDD__FrontLeftShaft.Trq[Nm]/1
  __TDD__FrontLeftShaft.Trq[Nm]/1 -> __TDO__FrontLeftShaft/1  "Trq[Nm]"
  RotSpdDifferentialOut[rad/s]___UNIQUE_1/1 -> __TDD__FrontLeftShaft.RotSpdDifferentialOut[rad/s]/1
  __TDD__FrontLeftShaft.RotSpdDifferentialOut[rad/s]/1 -> __TDO__FrontLeftShaft/2  "RotSpdDifferentialOut[rad/s]"
  RotAcc[rad/s**2]___UNIQUE_1/1 -> __TDD__FrontLeftShaft.RotAcc[rad/s**2]/1
  __TDD__FrontLeftShaft.RotAcc[rad/s**2]/1 -> __TDO__FrontLeftShaft/3  "RotAcc[rad/s**2]"
  DerivativeOfTrq_wrt_RotAng[Nm/rad]___UNIQUE_1/1 -> __TDD__FrontLeftShaft.DerivativeOfTrq_wrt_RotAng[Nm/rad]/1
  __TDD__FrontLeftShaft.DerivativeOfTrq_wrt_RotAng[Nm/rad]/1 -> __TDO__FrontLeftShaft/4  "DerivativeOfTrq_wrt_RotAng[Nm/rad]"
  DerivativeOfTrq_wrt_WheelSpd[Nm/(rad/s)]___UNIQUE_1/1 -> __TDD__FrontLeftShaft.DerivativeOfTrq_wrt_WheelSpd[Nm/(rad/s)]/1
  __TDD__FrontLeftShaft.DerivativeOfTrq_wrt_WheelSpd[Nm/(rad/s)]/1 -> __TDO__FrontLeftShaft/5  "DerivativeOfTrq_wrt_WheelSpd[Nm/(rad/s)]"
  AddInrt[kg*m**2]___UNIQUE_1/1 -> __TDD__FrontLeftShaft.AddInrt[kg*m**2]/1
  __TDD__FrontLeftShaft.AddInrt[kg*m**2]/1 -> __TDO__FrontLeftShaft/6  "AddInrt[kg*m**2]"
  FrictionTrq[Nm]___UNIQUE_1/1 -> __TDD__FrontLeftShaft.FrictionTrq[Nm]/1
  __TDD__FrontLeftShaft.FrictionTrq[Nm]/1 -> __TDO__FrontLeftShaft/7  "FrictionTrq[Nm]"
  __TDO__FrontLeftShaft/1 -> FrontLeftShaft___UNIQUE_1/1  "FrontLeftShaft"

== system PassengerCar/Vehicle/Drivetrain/DrivetrainPhysics/DrivetrainPhysicsOutputs/FrontRightShaftOutput/FrontRightShaftOutput ==
  Trq[Nm]___UNIQUE_1 : Inport  Description=|  PortDimensions=[1]
      | <name>Trq[Nm]</name>
      | <comment></comment>
  RotSpdDifferentialOut[rad/s]___UNIQUE_1 : Inport  Description=|  Port=2  PortDimensions=[1]
      | <name>RotSpdDifferentialOut[rad/s]</name>
      | <comment></comment>
  RotAcc[rad/s**2]___UNIQUE_1 : Inport  Description=|  Port=3  PortDimensions=[1]
      | <name>RotAcc[rad/s**2]</name>
      | <comment></comment>
  DerivativeOfTrq_wrt_RotAng[Nm/rad]___UNIQUE_1 : Inport  Description=|  Port=4  PortDimensions=[1]
      | <name>DerivativeOfTrq_wrt_RotAng[Nm/rad]</name>
      | <comment></comment>
  DerivativeOfTrq_wrt_WheelSpd[Nm/(rad/s)]___UNIQUE_1 : Inport  Description=|  Port=5  PortDimensions=[1]
      | <name>DerivativeOfTrq_wrt_WheelSpd[Nm/(rad/s)]</name>
      | <comment></comment>
  AddInrt[kg*m**2]___UNIQUE_1 : Inport  Description=|  Port=6  PortDimensions=[1]
      | <name>AddInrt[kg*m**2]</name>
      | <comment></comment>
  FrictionTrq[Nm]___UNIQUE_1 : Inport  Description=|  Port=7  PortDimensions=[1]
      | <name>FrictionTrq[Nm]</name>
      | <comment></comment>
  __TDD__FrontRightShaft.AddInrt[kg*m**2] : Demux  Outputs=[1]
  __TDD__FrontRightShaft.DerivativeOfTrq_wrt_RotAng[Nm/rad] : Demux  Outputs=[1]
  __TDD__FrontRightShaft.DerivativeOfTrq_wrt_WheelSpd[Nm/(rad/s)] : Demux  Outputs=[1]
  __TDD__FrontRightShaft.FrictionTrq[Nm] : Demux  Outputs=[1]
  __TDD__FrontRightShaft.RotAcc[rad/s**2] : Demux  Outputs=[1]
  __TDD__FrontRightShaft.RotSpdDifferentialOut[rad/s] : Demux  Outputs=[1]
  __TDD__FrontRightShaft.Trq[Nm] : Demux  Outputs=[1]
  __TDO__FrontRightShaft : BusCreator  Inputs=7
  FrontRightShaft___UNIQUE_1 : Outport  Description=|  PortDimensions=[7]  VectorParamsAs1DForOutWhenUnconnected=off
      | <name>Trq[Nm]</name>
      | <comment></comment>
  wires:
  Trq[Nm]___UNIQUE_1/1 -> __TDD__FrontRightShaft.Trq[Nm]/1
  __TDD__FrontRightShaft.Trq[Nm]/1 -> __TDO__FrontRightShaft/1  "Trq[Nm]"
  RotSpdDifferentialOut[rad/s]___UNIQUE_1/1 -> __TDD__FrontRightShaft.RotSpdDifferentialOut[rad/s]/1
  __TDD__FrontRightShaft.RotSpdDifferentialOut[rad/s]/1 -> __TDO__FrontRightShaft/2  "RotSpdDifferentialOut[rad/s]"
  RotAcc[rad/s**2]___UNIQUE_1/1 -> __TDD__FrontRightShaft.RotAcc[rad/s**2]/1
  __TDD__FrontRightShaft.RotAcc[rad/s**2]/1 -> __TDO__FrontRightShaft/3  "RotAcc[rad/s**2]"
  DerivativeOfTrq_wrt_RotAng[Nm/rad]___UNIQUE_1/1 -> __TDD__FrontRightShaft.DerivativeOfTrq_wrt_RotAng[Nm/rad]/1
  __TDD__FrontRightShaft.DerivativeOfTrq_wrt_RotAng[Nm/rad]/1 -> __TDO__FrontRightShaft/4  "DerivativeOfTrq_wrt_RotAng[Nm/rad]"
  DerivativeOfTrq_wrt_WheelSpd[Nm/(rad/s)]___UNIQUE_1/1 -> __TDD__FrontRightShaft.DerivativeOfTrq_wrt_WheelSpd[Nm/(rad/s)]/1
  __TDD__FrontRightShaft.DerivativeOfTrq_wrt_WheelSpd[Nm/(rad/s)]/1 -> __TDO__FrontRightShaft/5  "DerivativeOfTrq_wrt_WheelSpd[Nm/(rad/s)]"
  AddInrt[kg*m**2]___UNIQUE_1/1 -> __TDD__FrontRightShaft.AddInrt[kg*m**2]/1
  __TDD__FrontRightShaft.AddInrt[kg*m**2]/1 -> __TDO__FrontRightShaft/6  "AddInrt[kg*m**2]"
  FrictionTrq[Nm]___UNIQUE_1/1 -> __TDD__FrontRightShaft.FrictionTrq[Nm]/1
  __TDD__FrontRightShaft.FrictionTrq[Nm]/1 -> __TDO__FrontRightShaft/7  "FrictionTrq[Nm]"
  __TDO__FrontRightShaft/1 -> FrontRightShaft___UNIQUE_1/1  "FrontRightShaft"

== system PassengerCar/Vehicle/Drivetrain/DrivetrainPhysics/DrivetrainPhysicsOutputs/Rear2DifferentialOutput/Rear2DifferentialOutput ==
  InSpd[rad/s]___UNIQUE_1 : Inport  Description=|  PortDimensions=[1]
      | <name>InSpd[rad/s]</name>
      | <comment></comment>
  LeftOutCutTrq[Nm]___UNIQUE_1 : Inport  Description=|  Port=2  PortDimensions=[1]
      | <name>LeftOutCutTrq[Nm]</name>
      | <comment></comment>
  RightOutCutTrq[Nm]___UNIQUE_1 : Inport  Description=|  Port=3  PortDimensions=[1]
      | <name>RightOutCutTrq[Nm]</name>
      | <comment></comment>
  LossPower[W]___UNIQUE_1 : Inport  Description=|  Port=4  PortDimensions=[1]
      | <name>LossPower[W]</name>
      | <comment></comment>
  __TDD__Rear2Differential.InSpd[rad/s] : Demux  Outputs=[1]
  __TDD__Rear2Differential.LeftOutCutTrq[Nm] : Demux  Outputs=[1]
  __TDD__Rear2Differential.LossPower[W] : Demux  Outputs=[1]
  __TDD__Rear2Differential.RightOutCutTrq[Nm] : Demux  Outputs=[1]
  __TDO__Rear2Differential : BusCreator  Inputs=4
  Rear2Differential___UNIQUE_1 : Outport  Description=|  PortDimensions=[4]  VectorParamsAs1DForOutWhenUnconnected=off
      | <name>InSpd[rad/s]</name>
      | <comment></comment>
  wires:
  InSpd[rad/s]___UNIQUE_1/1 -> __TDD__Rear2Differential.InSpd[rad/s]/1
  __TDD__Rear2Differential.InSpd[rad/s]/1 -> __TDO__Rear2Differential/1  "InSpd[rad/s]"
  LeftOutCutTrq[Nm]___UNIQUE_1/1 -> __TDD__Rear2Differential.LeftOutCutTrq[Nm]/1
  __TDD__Rear2Differential.LeftOutCutTrq[Nm]/1 -> __TDO__Rear2Differential/2  "LeftOutCutTrq[Nm]"
  RightOutCutTrq[Nm]___UNIQUE_1/1 -> __TDD__Rear2Differential.RightOutCutTrq[Nm]/1
  __TDD__Rear2Differential.RightOutCutTrq[Nm]/1 -> __TDO__Rear2Differential/3  "RightOutCutTrq[Nm]"
  LossPower[W]___UNIQUE_1/1 -> __TDD__Rear2Differential.LossPower[W]/1
  __TDD__Rear2Differential.LossPower[W]/1 -> __TDO__Rear2Differential/4  "LossPower[W]"
  __TDO__Rear2Differential/1 -> Rear2Differential___UNIQUE_1/1  "Rear2Differential"

== system PassengerCar/Vehicle/Drivetrain/DrivetrainPhysics/DrivetrainPhysicsOutputs/Rear2LeftShaftOutput/Rear2LeftShaftOutput ==
  Trq[Nm]___UNIQUE_1 : Inport  Description=|  PortDimensions=[1]
      | <name>Trq[Nm]</name>
      | <comment></comment>
  RotSpdDifferentialOut[rad/s]___UNIQUE_1 : Inport  Description=|  Port=2  PortDimensions=[1]
      | <name>RotSpdDifferentialOut[rad/s]</name>
      | <comment></comment>
  RotAcc[rad/s**2]___UNIQUE_1 : Inport  Description=|  Port=3  PortDimensions=[1]
      | <name>RotAcc[rad/s**2]</name>
      | <comment></comment>
  DerivativeOfTrq_wrt_RotAng[Nm/rad]___UNIQUE_1 : Inport  Description=|  Port=4  PortDimensions=[1]
      | <name>DerivativeOfTrq_wrt_RotAng[Nm/rad]</name>
      | <comment></comment>
  DerivativeOfTrq_wrt_WheelSpd[Nm/(rad/s)]___UNIQUE_1 : Inport  Description=|  Port=5  PortDimensions=[1]
      | <name>DerivativeOfTrq_wrt_WheelSpd[Nm/(rad/s)]</name>
      | <comment></comment>
  AddInrt[kg*m**2]___UNIQUE_1 : Inport  Description=|  Port=6  PortDimensions=[1]
      | <name>AddInrt[kg*m**2]</name>
      | <comment></comment>
  FrictionTrq[Nm]___UNIQUE_1 : Inport  Description=|  Port=7  PortDimensions=[1]
      | <name>FrictionTrq[Nm]</name>
      | <comment></comment>
  __TDD__Rear2LeftShaft.AddInrt[kg*m**2] : Demux  Outputs=[1]
  __TDD__Rear2LeftShaft.DerivativeOfTrq_wrt_RotAng[Nm/rad] : Demux  Outputs=[1]
  __TDD__Rear2LeftShaft.DerivativeOfTrq_wrt_WheelSpd[Nm/(rad/s)] : Demux  Outputs=[1]
  __TDD__Rear2LeftShaft.FrictionTrq[Nm] : Demux  Outputs=[1]
  __TDD__Rear2LeftShaft.RotAcc[rad/s**2] : Demux  Outputs=[1]
  __TDD__Rear2LeftShaft.RotSpdDifferentialOut[rad/s] : Demux  Outputs=[1]
  __TDD__Rear2LeftShaft.Trq[Nm] : Demux  Outputs=[1]
  __TDO__Rear2LeftShaft : BusCreator  Inputs=7
  Rear2LeftShaft___UNIQUE_1 : Outport  Description=|  PortDimensions=[7]  VectorParamsAs1DForOutWhenUnconnected=off
      | <name>Trq[Nm]</name>
      | <comment></comment>
  wires:
  Trq[Nm]___UNIQUE_1/1 -> __TDD__Rear2LeftShaft.Trq[Nm]/1
  __TDD__Rear2LeftShaft.Trq[Nm]/1 -> __TDO__Rear2LeftShaft/1  "Trq[Nm]"
  RotSpdDifferentialOut[rad/s]___UNIQUE_1/1 -> __TDD__Rear2LeftShaft.RotSpdDifferentialOut[rad/s]/1
  __TDD__Rear2LeftShaft.RotSpdDifferentialOut[rad/s]/1 -> __TDO__Rear2LeftShaft/2  "RotSpdDifferentialOut[rad/s]"
  RotAcc[rad/s**2]___UNIQUE_1/1 -> __TDD__Rear2LeftShaft.RotAcc[rad/s**2]/1
  __TDD__Rear2LeftShaft.RotAcc[rad/s**2]/1 -> __TDO__Rear2LeftShaft/3  "RotAcc[rad/s**2]"
  DerivativeOfTrq_wrt_RotAng[Nm/rad]___UNIQUE_1/1 -> __TDD__Rear2LeftShaft.DerivativeOfTrq_wrt_RotAng[Nm/rad]/1
  __TDD__Rear2LeftShaft.DerivativeOfTrq_wrt_RotAng[Nm/rad]/1 -> __TDO__Rear2LeftShaft/4  "DerivativeOfTrq_wrt_RotAng[Nm/rad]"
  DerivativeOfTrq_wrt_WheelSpd[Nm/(rad/s)]___UNIQUE_1/1 -> __TDD__Rear2LeftShaft.DerivativeOfTrq_wrt_WheelSpd[Nm/(rad/s)]/1
  __TDD__Rear2LeftShaft.DerivativeOfTrq_wrt_WheelSpd[Nm/(rad/s)]/1 -> __TDO__Rear2LeftShaft/5  "DerivativeOfTrq_wrt_WheelSpd[Nm/(rad/s)]"
  AddInrt[kg*m**2]___UNIQUE_1/1 -> __TDD__Rear2LeftShaft.AddInrt[kg*m**2]/1
  __TDD__Rear2LeftShaft.AddInrt[kg*m**2]/1 -> __TDO__Rear2LeftShaft/6  "AddInrt[kg*m**2]"
  FrictionTrq[Nm]___UNIQUE_1/1 -> __TDD__Rear2LeftShaft.FrictionTrq[Nm]/1
  __TDD__Rear2LeftShaft.FrictionTrq[Nm]/1 -> __TDO__Rear2LeftShaft/7  "FrictionTrq[Nm]"
  __TDO__Rear2LeftShaft/1 -> Rear2LeftShaft___UNIQUE_1/1  "Rear2LeftShaft"

== system PassengerCar/Vehicle/Drivetrain/DrivetrainPhysics/DrivetrainPhysicsOutputs/Rear2RightShaftOutput/Rear2RightShaftOutput ==
  Trq[Nm]___UNIQUE_1 : Inport  Description=|  PortDimensions=[1]
      | <name>Trq[Nm]</name>
      | <comment></comment>
  RotSpdDifferentialOut[rad/s]___UNIQUE_1 : Inport  Description=|  Port=2  PortDimensions=[1]
      | <name>RotSpdDifferentialOut[rad/s]</name>
      | <comment></comment>
  RotAcc[rad/s**2]___UNIQUE_1 : Inport  Description=|  Port=3  PortDimensions=[1]
      | <name>RotAcc[rad/s**2]</name>
      | <comment></comment>
  DerivativeOfTrq_wrt_RotAng[Nm/rad]___UNIQUE_1 : Inport  Description=|  Port=4  PortDimensions=[1]
      | <name>DerivativeOfTrq_wrt_RotAng[Nm/rad]</name>
      | <comment></comment>
  DerivativeOfTrq_wrt_WheelSpd[Nm/(rad/s)]___UNIQUE_1 : Inport  Description=|  Port=5  PortDimensions=[1]
      | <name>DerivativeOfTrq_wrt_WheelSpd[Nm/(rad/s)]</name>
      | <comment></comment>
  AddInrt[kg*m**2]___UNIQUE_1 : Inport  Description=|  Port=6  PortDimensions=[1]
      | <name>AddInrt[kg*m**2]</name>
      | <comment></comment>
  FrictionTrq[Nm]___UNIQUE_1 : Inport  Description=|  Port=7  PortDimensions=[1]
      | <name>FrictionTrq[Nm]</name>
      | <comment></comment>
  __TDD__Rear2RightShaft.AddInrt[kg*m**2] : Demux  Outputs=[1]
  __TDD__Rear2RightShaft.DerivativeOfTrq_wrt_RotAng[Nm/rad] : Demux  Outputs=[1]
  __TDD__Rear2RightShaft.DerivativeOfTrq_wrt_WheelSpd[Nm/(rad/s)] : Demux  Outputs=[1]
  __TDD__Rear2RightShaft.FrictionTrq[Nm] : Demux  Outputs=[1]
  __TDD__Rear2RightShaft.RotAcc[rad/s**2] : Demux  Outputs=[1]
  __TDD__Rear2RightShaft.RotSpdDifferentialOut[rad/s] : Demux  Outputs=[1]
  __TDD__Rear2RightShaft.Trq[Nm] : Demux  Outputs=[1]
  __TDO__Rear2RightShaft : BusCreator  Inputs=7
  Rear2RightShaft___UNIQUE_1 : Outport  Description=|  PortDimensions=[7]  VectorParamsAs1DForOutWhenUnconnected=off
      | <name>Trq[Nm]</name>
      | <comment></comment>
  wires:
  Trq[Nm]___UNIQUE_1/1 -> __TDD__Rear2RightShaft.Trq[Nm]/1
  __TDD__Rear2RightShaft.Trq[Nm]/1 -> __TDO__Rear2RightShaft/1  "Trq[Nm]"
  RotSpdDifferentialOut[rad/s]___UNIQUE_1/1 -> __TDD__Rear2RightShaft.RotSpdDifferentialOut[rad/s]/1
  __TDD__Rear2RightShaft.RotSpdDifferentialOut[rad/s]/1 -> __TDO__Rear2RightShaft/2  "RotSpdDifferentialOut[rad/s]"
  RotAcc[rad/s**2]___UNIQUE_1/1 -> __TDD__Rear2RightShaft.RotAcc[rad/s**2]/1
  __TDD__Rear2RightShaft.RotAcc[rad/s**2]/1 -> __TDO__Rear2RightShaft/3  "RotAcc[rad/s**2]"
  DerivativeOfTrq_wrt_RotAng[Nm/rad]___UNIQUE_1/1 -> __TDD__Rear2RightShaft.DerivativeOfTrq_wrt_RotAng[Nm/rad]/1
  __TDD__Rear2RightShaft.DerivativeOfTrq_wrt_RotAng[Nm/rad]/1 -> __TDO__Rear2RightShaft/4  "DerivativeOfTrq_wrt_RotAng[Nm/rad]"
  DerivativeOfTrq_wrt_WheelSpd[Nm/(rad/s)]___UNIQUE_1/1 -> __TDD__Rear2RightShaft.DerivativeOfTrq_wrt_WheelSpd[Nm/(rad/s)]/1
  __TDD__Rear2RightShaft.DerivativeOfTrq_wrt_WheelSpd[Nm/(rad/s)]/1 -> __TDO__Rear2RightShaft/5  "DerivativeOfTrq_wrt_WheelSpd[Nm/(rad/s)]"
  AddInrt[kg*m**2]___UNIQUE_1/1 -> __TDD__Rear2RightShaft.AddInrt[kg*m**2]/1
  __TDD__Rear2RightShaft.AddInrt[kg*m**2]/1 -> __TDO__Rear2RightShaft/6  "AddInrt[kg*m**2]"
  FrictionTrq[Nm]___UNIQUE_1/1 -> __TDD__Rear2RightShaft.FrictionTrq[Nm]/1
  __TDD__Rear2RightShaft.FrictionTrq[Nm]/1 -> __TDO__Rear2RightShaft/7  "FrictionTrq[Nm]"
  __TDO__Rear2RightShaft/1 -> Rear2RightShaft___UNIQUE_1/1  "Rear2RightShaft"

== system PassengerCar/Vehicle/Drivetrain/DrivetrainPhysics/DrivetrainPhysicsOutputs/Rear3DifferentialOutput/Rear3DifferentialOutput ==
  InSpd[rad/s]___UNIQUE_1 : Inport  Description=|  PortDimensions=[1]
      | <name>InSpd[rad/s]</name>
      | <comment></comment>
  LeftOutCutTrq[Nm]___UNIQUE_1 : Inport  Description=|  Port=2  PortDimensions=[1]
      | <name>LeftOutCutTrq[Nm]</name>
      | <comment></comment>
  RightOutCutTrq[Nm]___UNIQUE_1 : Inport  Description=|  Port=3  PortDimensions=[1]
      | <name>RightOutCutTrq[Nm]</name>
      | <comment></comment>
  LossPower[W]___UNIQUE_1 : Inport  Description=|  Port=4  PortDimensions=[1]
      | <name>LossPower[W]</name>
      | <comment></comment>
  __TDD__Rear3Differential.InSpd[rad/s] : Demux  Outputs=[1]
  __TDD__Rear3Differential.LeftOutCutTrq[Nm] : Demux  Outputs=[1]
  __TDD__Rear3Differential.LossPower[W] : Demux  Outputs=[1]
  __TDD__Rear3Differential.RightOutCutTrq[Nm] : Demux  Outputs=[1]
  __TDO__Rear3Differential : BusCreator  Inputs=4
  Rear3Differential___UNIQUE_1 : Outport  Description=|  PortDimensions=[4]  VectorParamsAs1DForOutWhenUnconnected=off
      | <name>InSpd[rad/s]</name>
      | <comment></comment>
  wires:
  InSpd[rad/s]___UNIQUE_1/1 -> __TDD__Rear3Differential.InSpd[rad/s]/1
  __TDD__Rear3Differential.InSpd[rad/s]/1 -> __TDO__Rear3Differential/1  "InSpd[rad/s]"
  LeftOutCutTrq[Nm]___UNIQUE_1/1 -> __TDD__Rear3Differential.LeftOutCutTrq[Nm]/1
  __TDD__Rear3Differential.LeftOutCutTrq[Nm]/1 -> __TDO__Rear3Differential/2  "LeftOutCutTrq[Nm]"
  RightOutCutTrq[Nm]___UNIQUE_1/1 -> __TDD__Rear3Differential.RightOutCutTrq[Nm]/1
  __TDD__Rear3Differential.RightOutCutTrq[Nm]/1 -> __TDO__Rear3Differential/3  "RightOutCutTrq[Nm]"
  LossPower[W]___UNIQUE_1/1 -> __TDD__Rear3Differential.LossPower[W]/1
  __TDD__Rear3Differential.LossPower[W]/1 -> __TDO__Rear3Differential/4  "LossPower[W]"
  __TDO__Rear3Differential/1 -> Rear3Differential___UNIQUE_1/1  "Rear3Differential"

== system PassengerCar/Vehicle/Drivetrain/DrivetrainPhysics/DrivetrainPhysicsOutputs/Rear3LeftShaftOutput/Rear3LeftShaftOutput ==
  Trq[Nm]___UNIQUE_1 : Inport  Description=|  PortDimensions=[1]
      | <name>Trq[Nm]</name>
      | <comment></comment>
  RotSpdDifferentialOut[rad/s]___UNIQUE_1 : Inport  Description=|  Port=2  PortDimensions=[1]
      | <name>RotSpdDifferentialOut[rad/s]</name>
      | <comment></comment>
  RotAcc[rad/s**2]___UNIQUE_1 : Inport  Description=|  Port=3  PortDimensions=[1]
      | <name>RotAcc[rad/s**2]</name>
      | <comment></comment>
  DerivativeOfTrq_wrt_RotAng[Nm/rad]___UNIQUE_1 : Inport  Description=|  Port=4  PortDimensions=[1]
      | <name>DerivativeOfTrq_wrt_RotAng[Nm/rad]</name>
      | <comment></comment>
  DerivativeOfTrq_wrt_WheelSpd[Nm/(rad/s)]___UNIQUE_1 : Inport  Description=|  Port=5  PortDimensions=[1]
      | <name>DerivativeOfTrq_wrt_WheelSpd[Nm/(rad/s)]</name>
      | <comment></comment>
  AddInrt[kg*m**2]___UNIQUE_1 : Inport  Description=|  Port=6  PortDimensions=[1]
      | <name>AddInrt[kg*m**2]</name>
      | <comment></comment>
  FrictionTrq[Nm]___UNIQUE_1 : Inport  Description=|  Port=7  PortDimensions=[1]
      | <name>FrictionTrq[Nm]</name>
      | <comment></comment>
  __TDD__Rear3LeftShaft.AddInrt[kg*m**2] : Demux  Outputs=[1]
  __TDD__Rear3LeftShaft.DerivativeOfTrq_wrt_RotAng[Nm/rad] : Demux  Outputs=[1]
  __TDD__Rear3LeftShaft.DerivativeOfTrq_wrt_WheelSpd[Nm/(rad/s)] : Demux  Outputs=[1]
  __TDD__Rear3LeftShaft.FrictionTrq[Nm] : Demux  Outputs=[1]
  __TDD__Rear3LeftShaft.RotAcc[rad/s**2] : Demux  Outputs=[1]
  __TDD__Rear3LeftShaft.RotSpdDifferentialOut[rad/s] : Demux  Outputs=[1]
  __TDD__Rear3LeftShaft.Trq[Nm] : Demux  Outputs=[1]
  __TDO__Rear3LeftShaft : BusCreator  Inputs=7
  Rear3LeftShaft___UNIQUE_1 : Outport  Description=|  PortDimensions=[7]  VectorParamsAs1DForOutWhenUnconnected=off
      | <name>Trq[Nm]</name>
      | <comment></comment>
  wires:
  Trq[Nm]___UNIQUE_1/1 -> __TDD__Rear3LeftShaft.Trq[Nm]/1
  __TDD__Rear3LeftShaft.Trq[Nm]/1 -> __TDO__Rear3LeftShaft/1  "Trq[Nm]"
  RotSpdDifferentialOut[rad/s]___UNIQUE_1/1 -> __TDD__Rear3LeftShaft.RotSpdDifferentialOut[rad/s]/1
  __TDD__Rear3LeftShaft.RotSpdDifferentialOut[rad/s]/1 -> __TDO__Rear3LeftShaft/2  "RotSpdDifferentialOut[rad/s]"
  RotAcc[rad/s**2]___UNIQUE_1/1 -> __TDD__Rear3LeftShaft.RotAcc[rad/s**2]/1
  __TDD__Rear3LeftShaft.RotAcc[rad/s**2]/1 -> __TDO__Rear3LeftShaft/3  "RotAcc[rad/s**2]"
  DerivativeOfTrq_wrt_RotAng[Nm/rad]___UNIQUE_1/1 -> __TDD__Rear3LeftShaft.DerivativeOfTrq_wrt_RotAng[Nm/rad]/1
  __TDD__Rear3LeftShaft.DerivativeOfTrq_wrt_RotAng[Nm/rad]/1 -> __TDO__Rear3LeftShaft/4  "DerivativeOfTrq_wrt_RotAng[Nm/rad]"
  DerivativeOfTrq_wrt_WheelSpd[Nm/(rad/s)]___UNIQUE_1/1 -> __TDD__Rear3LeftShaft.DerivativeOfTrq_wrt_WheelSpd[Nm/(rad/s)]/1
  __TDD__Rear3LeftShaft.DerivativeOfTrq_wrt_WheelSpd[Nm/(rad/s)]/1 -> __TDO__Rear3LeftShaft/5  "DerivativeOfTrq_wrt_WheelSpd[Nm/(rad/s)]"
  AddInrt[kg*m**2]___UNIQUE_1/1 -> __TDD__Rear3LeftShaft.AddInrt[kg*m**2]/1
  __TDD__Rear3LeftShaft.AddInrt[kg*m**2]/1 -> __TDO__Rear3LeftShaft/6  "AddInrt[kg*m**2]"
  FrictionTrq[Nm]___UNIQUE_1/1 -> __TDD__Rear3LeftShaft.FrictionTrq[Nm]/1
  __TDD__Rear3LeftShaft.FrictionTrq[Nm]/1 -> __TDO__Rear3LeftShaft/7  "FrictionTrq[Nm]"
  __TDO__Rear3LeftShaft/1 -> Rear3LeftShaft___UNIQUE_1/1  "Rear3LeftShaft"
